simulink model "testrig_Bus_Makhulu_Parts"  (R2026a)
settings: Solver=VariableStepAuto  EnableMultiTasking=on
undefined symbols (not defined in the file): X, Y, Z
libraries: sm_lib x9, Bus_Makhulu_Parts x6, Passenger_Human x4, nesl_utility x1
Description:
  | Copyright 2020-2026 The MathWorks, Inc.
settings Model: Creator=smiller  LastModifiedBy=smiller
settings DataIOCC: SignalLoggingName=logsout_testrig_Bus_Makhulu_Parts
settings SimscapeCC: SimscapeNominalValues="[{\"value\":\"10\",\"unit\":\"V\"},{\"value\":\"1\",\"unit\":\"A\"},{\"value\":\"10\",\"unit\":\"N*m\"},{\"value\":\"10\",\"unit\":\"bar\"},{\"value\":\"100\",\"unit\":\"kJ/kg\"},{\"value\":\"1\",\"unit\":\"kW\"},{\"value\":\"300\",\"unit\":\"K\"},{\"value\":\"100\",\"unit\":\"cm^3/s\"},{\"value\":\"1\",\"unit\":\"kN\"},{\"value\":\"1\",\"unit\":\"g/cm^3\"},{\"value\":\"1\",\"unit\":\"l\"},{\"value\":\"1\",\"unit\":\"cm^2\"},{\"value\":\"60\",\"unit\":\"Hz\"}]"  SimscapeLogName=simlog_testrig_Bus_Makhulu_Parts
settings ConfigurationSet: Description=SimMechanics 2G
settings ExplorerConfigSet: InternalSimMechanicsExplorerSettings="<ExplorerConfiguration><canonicalview>default</canonicalview><AnimationSetting><BasePlaybackSpeed>1.0</BasePlaybackSpeed><PlaybackSpeedFactor>1.0</PlaybackSpeedFactor></AnimationSetting><TilePanel><TileInfo><Tiles Columns=\"4\" Count=\"6\" Rows=\"3\"><Column Weight=\"0.3469\"/><Column Weight=\"0.3469\"/><Column Weight=\"0.1531\"/><Column Weight=\"0.1531\"/><Row Weight=\"0.5025\"/><Row Weight=\"0.2487\"/><Row Weight=\"0.2487\"/><Tile Height=\"1\" Width=\"1\" X=\"0\" Y=\"0\"/><Tile Height=\"1\" Width=\"1\" X=\"1\" Y=\"0\"/><Tile Height=\"1\" Width=\"2\" X=\"0\" Y=\"1\"/><Tile Height=\"1\" Width=\"2\" X=\"0\" Y=\"2\"/><Tile Height=\"3\" Width=\"1\" X=\"2\" Y=\"0\"/><Tile Height=\"3\" Width=\"1\" X=\"3\" Y=\"0\"/></Tiles></TileInfo><SceneInfo><SceneViewer><BGColor><R>1</R><G>1</G><B>1</B></BGColor><Camera><DoPerspective>off</DoPerspective><Position><X>2.89597907673196531</X><Y>-0.00109799404478061469</Y><Z>1.33429143595940403</Z></Position><Center><X>-3.84443919785476673</X><Y>-0.00109799404478061469</Y><Z>1.33429143595940403</Z></Center><Up><X>-0</X><Y>0</Y><Z>1</Z></Up><ViewLimDist>1</ViewLimDist><YLim>1.37425733566284181</YLim><XLim>1.46067108293575876</XLim></Camera></SceneViewer><SceneViewer><BGColor><R>1</R><G>1</G><B>1</B></BGColor><Camera><DoPerspective>off</DoPerspective><Position><X>-10.8501736304465091</X><Y>-0.00109795652245203712</Y><Z>1.33429143595940225</Z></Position><Center><X>-3.84443855103689636</X><Y>-0.00109795652245203712</Y><Z>1.33429143595940225</Z></Center><Up><X>0</X><Y>0</Y><Z>1</Z></Up><ViewLimDist>1</ViewLimDist><YLim>1.37425733566284181</YLim><XLim>1.46067108293575876</XLim></Camera></SceneViewer><SceneViewer><BGColor><R>1</R><G>1</G><B>1</B></BGColor><Camera><DoPerspective>off</DoPerspective><Position><X>-3.84443881153779143</X><Y>-6.9199634574691915</Y><Z>1.33429143595940314</Z></Position><Center><X>-3.84443881153779143</X><Y>-0.00109763641691196234</Y><Z>1.33429143595940314</Z></Center><Up><X>0</X><Y>-0</Y><Z>1</Z></Up><ViewLimDist>1</ViewLimDist><YLim>1.37425733566284181</YLim><XLim>6.00243803221332239</XLim></Camera></SceneViewer><SceneViewer><BGColor><R>1</R><G>1</G><B>1</B></BGColor><Camera><DoPerspective>off</DoPerspective><Position><X>-3.84443881153779055</X><Y>6.9177671418572757</Y><Z>1.33429143595940136</Z></Position><Center><X>-3.84443881153779055</X><Y>-0.00109815741870300521</Y><Z>1.33429143595940136</Z></Center><Up><X>0</X><Y>0</Y><Z>1</Z></Up><ViewLimDist>1</ViewLimDist><YLim>1.37425733566284181</YLim><XLim>6.00243803221332239</XLim></Camera></SceneViewer><SceneViewer><BGColor><R>1</R><G>1</G><B>1</B></BGColor><Camera><DoPerspective>off</DoPerspective><Position><X>-3.84496310619994697</X><Y>0.00593013000974051963</Y><Z>8.58263582377032996</Z></Position><Center><X>-3.84496310619994697</X><Y>0.00593013000974051963</Y><Z>1.33429140250232159</Z></Center><Up><X>0.999999127014181366</X><Y>-0.00132135191201654401</Y><Z>0</Z></Up><ViewLimDist>1</ViewLimDist><YLim>5.96790659427642822</YLim><XLim>1.37351820109477596</XLim></Camera></SceneViewer><SceneViewer><BGColor><R>1</R><G>1</G><B>1</B></BGColor><Camera><DoPerspective>off</DoPerspective><Position><X>-3.84487511554848593</X><Y>-0.0069608981245425916</Y><Z>-5.25447968591559</Z></Position><Center><X>-3.84487511554848593</X><Y>-0.0069608981245425916</Y><Z>1.3342916573167356</Z></Center><Up><X>0.999999392465900749</X><Y>0.00110230115204205253</Y><Z>0</Z></Up><ViewLimDist>1</ViewLimDist><YLim>5.96775483131408713</YLim><XLim>1.37348327273459891</XLim></Camera></SceneViewer></SceneInfo></TilePanel><MechEditorPanel><Cameras/><GfxPanelCameraMap/><VideoCreator><PlaybackSpeedRatio>1.0</PlaybackSpeedRatio><FrameRate>30</FrameRate><VideoFormat>Motion JPEG AVI</VideoFormat><FrameSize>auto</FrameSize></VideoCreator></MechEditorPanel></ExplorerConfiguration>"

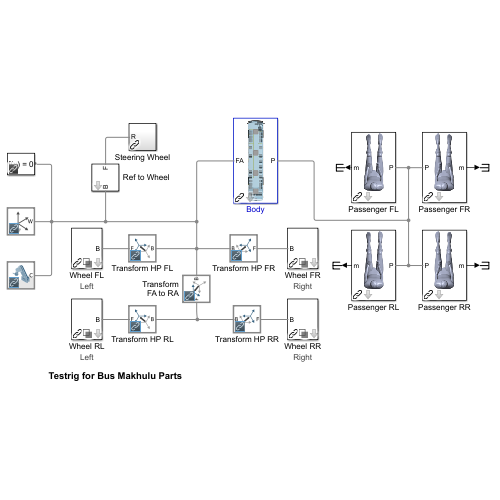
[thumbnail: Simulink's stored preview of the top-level diagram]
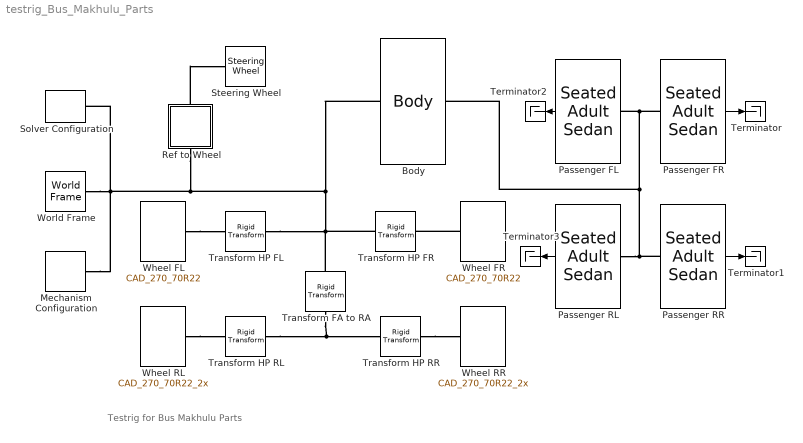
== system testrig_Bus_Makhulu_Parts ==
  note: Testrig for Bus Makhulu Parts
  Body : Bus_Makhulu_Parts/Body  body_offset=[0 0 0]  body_orient=[0 0 0]  body_clr=[0.55 0.85 1]  body_opc=1  glass_opc=BodyGeometry.GlassOpacity.Value
  Mechanism Configuration : sm_lib/Utilities/Mechanism Configuration  UniformGravity=Constant  GravityVector=[0 0 -9.80665]  GravityVectorUnits=m/s^2  LinearizationDelta=0.001  JointModeTransitionNonlinearIterations=2
  Passenger FL : Passenger_Human/Seated Adult Sedan  VariantControl=Variant1  hp_human=[-0.47 0.6 1.34]  rpy_human=[0 15 -90]  rho_human=Vehicle.Chassis.Body.Passenger.FL.rho.Value  human_clr=[0.792156862745098 0.819607843137255 0.933333333333333]  human_opc=1
  Passenger FR : Passenger_Human/Seated Adult Sedan  VariantControl=Variant1  hp_human=[-0.98 -0.6 1.34]  rpy_human=[0 15 90]  rho_human=Vehicle.Chassis.Body.Passenger.FL.rho.Value  human_clr=[0.792156862745098 0.819607843137255 0.933333333333333]  human_opc=1
  Passenger RL : Passenger_Human/Seated Adult Sedan  VariantControl=Variant1  hp_human=[-2.03 0.755 1.2]  rpy_human=[0 15 180]  rho_human=Vehicle.Chassis.Body.Passenger.FL.rho.Value  human_clr=[0.792156862745098 0.819607843137255 0.933333333333333]  human_opc=1
  Passenger RR : Passenger_Human/Seated Adult Sedan  VariantControl=Variant1  hp_human=[-3.05 -0.77 1.2]  rpy_human=[0 15 0]  rho_human=Vehicle.Chassis.Body.Passenger.FL.rho.Value  human_clr=[0.792156862745098 0.819607843137255 0.933333333333333]  human_opc=1
  Ref to Wheel : Subsystem  mask{hp_wheel=[1.2610308+0.01 0.55801 1.2685808], wheel_axis_incl=45.2*pi/180}
      mask prompts: hp_wheel "HP Steering Wheel [x y z] (m)"; wheel_axis_incl "Steering Inclination Angle (rad)"
  Solver Configuration : nesl_utility/Solver Configuration  PhysicalDomain=network_engine_domain  SubClassName=solver  LeftPortType=input  RightPortType=generic  Tones=[]  Harmonics=[]  SimulateNoise=off  Profile=off  UseLocalSampling=off  EnableSwitchedLinearOptims=on  FrequencyDomain=off  UseCCode=off  RelTol=0.001  AbsTol=1e-06  MinStep=1e-09  ToWorkspace=off  RevertToSquareIcSolve=off  NumHomotopyIterations=100  PhasorMode=off  PhasorModeNumHarmonics=1  ConsistencySolver=NEWTON_FTOL  CanonicalOrdering=UNORDERED  OptimizeIntermediates=UNOPTIMIZED  IndexReductionMethod=DerivativeReplacement  DoDC=off  ResidualTolerance=1e-09  ConsistencyTolSource=GLOBAL  ConsistencyAbsTol=0.001  ConsistencyRelTol=0.001  ConsistencyTolFactor=0.001  UseLocalSolver=off  LocalSolverChoice=NE_BACKWARD_EULER_ADVANCER  ResolveIndetEquations=on  FunctionEvalNumThread=1  LocalSolverSampleTime=0.001  DoFixedCost=off  MaxNonlinIter=3  MaxModeIter=2  ComputeImpulses=off  ImpulseIterations=2  LinearAlgebra=Sparse  LinearAlgebraNumThread=0  EquationFormulation=NE_TIME_EF  DelaysMemoryBudget=1024  AutomaticFiltering=on  FilteringTimeConstant=0.001  PartitionStorageMethod=AS_NEEDED  PartitionMemoryBudget=1024  PartitionMethod=FAST  MultibodyUseLocalSolver=off  MultibodyLocalSolverChoice=ODE1  MultibodyLocalSolverSampleTime=0.001
  Steering Wheel : Bus_Makhulu_Parts/Steering Wheel  SystemSampleTime=-1  VariantActivationTime=update diagram  EmptyChoice=off  PassThrough=off  PassThroughVariantControl=(default)  EmptyChoiceVariantControl=(default)  AllowFlexibleInterface=on  Latency=0  AutoFrameSizeCalculation=off
  Terminator{,1..3} (4 alike) : Terminator
  Transform FA to RA : sm_lib/Frames and Transforms/Rigid Transform  RotationMethod=None  FollAlignAxisA=+X  BaseAlignAxisA=+Y  FollAlignAxisB=+Y  BaseAlignAxisB=+Z  RotationStandardAxis=+Z  RotationAngle=0.0  RotationAngleUnits=deg  RotationArbitraryAxis=[0 0 1]  RotationSequenceAxes=FollowerAxes  RotationSequence=XYX  RotationSequenceAngles=[0 0 0]  RotationSequenceAnglesUnits=deg  RotationMatrix=[1 0 0; 0 1 0; 0 0 1]  Quaternion=[1 0 0 0]  TranslationMethod=StandardAxis  TranslationCartesianOffset=[0 0 0]  TranslationCartesianOffsetUnits=m  TranslationStandardAxis=+X  TranslationStandardOffset=-6.781616  TranslationStandardOffsetUnits=m  TranslationROffset=0  TranslationROffsetUnits=m  TranslationThetaOffset=0  TranslationThetaOffsetUnits=deg  TranslationZOffset=0  TranslationZOffsetUnits=m
  Transform HP FL : sm_lib/Frames and Transforms/Rigid Transform  RotationMethod=StandardAxis  FollAlignAxisA=+X  BaseAlignAxisA=+Y  FollAlignAxisB=+Y  BaseAlignAxisB=+Z  RotationStandardAxis=+X  RotationAngle=-90  RotationAngleUnits=deg  RotationArbitraryAxis=[0 0 1]  RotationSequenceAxes=FollowerAxes  RotationSequence=XYX  RotationSequenceAngles=[0 0 0]  RotationSequenceAnglesUnits=deg  RotationMatrix=[1 0 0; 0 1 0; 0 0 1]  Quaternion=[1 0 0 0]  TranslationMethod=Cartesian  TranslationCartesianOffset=[0 0.9829099 0.4613615]  TranslationCartesianOffsetUnits=m  TranslationStandardAxis=+Z  TranslationStandardOffset=0  TranslationStandardOffsetUnits=m  TranslationROffset=0  TranslationROffsetUnits=m  TranslationThetaOffset=0  TranslationThetaOffsetUnits=deg  TranslationZOffset=0  TranslationZOffsetUnits=m
  Transform HP FR : sm_lib/Frames and Transforms/Rigid Transform  RotationMethod=StandardAxis  FollAlignAxisA=+X  BaseAlignAxisA=+Y  FollAlignAxisB=+Y  BaseAlignAxisB=+Z  RotationStandardAxis=+X  RotationAngle=-90  RotationAngleUnits=deg  RotationArbitraryAxis=[0 0 1]  RotationSequenceAxes=FollowerAxes  RotationSequence=XYX  RotationSequenceAngles=[0 0 0]  RotationSequenceAnglesUnits=deg  RotationMatrix=[1 0 0; 0 1 0; 0 0 1]  Quaternion=[1 0 0 0]  TranslationMethod=Cartesian  TranslationCartesianOffset=[0 -0.9829099 0.4613615]  TranslationCartesianOffsetUnits=m  TranslationStandardAxis=+Z  TranslationStandardOffset=0  TranslationStandardOffsetUnits=m  TranslationROffset=0  TranslationROffsetUnits=m  TranslationThetaOffset=0  TranslationThetaOffsetUnits=deg  TranslationZOffset=0  TranslationZOffsetUnits=m
  Transform HP RL : sm_lib/Frames and Transforms/Rigid Transform  RotationMethod=StandardAxis  FollAlignAxisA=+X  BaseAlignAxisA=+Y  FollAlignAxisB=+Y  BaseAlignAxisB=+Z  RotationStandardAxis=+X  RotationAngle=-90  RotationAngleUnits=deg  RotationArbitraryAxis=[0 0 1]  RotationSequenceAxes=FollowerAxes  RotationSequence=XYX  RotationSequenceAngles=[0 0 0]  RotationSequenceAnglesUnits=deg  RotationMatrix=[1 0 0; 0 1 0; 0 0 1]  Quaternion=[1 0 0 0]  TranslationMethod=Cartesian  TranslationCartesianOffset="[0 0.838344+0.1359705  0.4613615]"  TranslationCartesianOffsetUnits=m  TranslationStandardAxis=+Z  TranslationStandardOffset=0  TranslationStandardOffsetUnits=m  TranslationROffset=0  TranslationROffsetUnits=m  TranslationThetaOffset=0  TranslationThetaOffsetUnits=deg  TranslationZOffset=0  TranslationZOffsetUnits=m
  Transform HP RR : sm_lib/Frames and Transforms/Rigid Transform  RotationMethod=StandardAxis  FollAlignAxisA=+X  BaseAlignAxisA=+Y  FollAlignAxisB=+Y  BaseAlignAxisB=+Z  RotationStandardAxis=+X  RotationAngle=-90  RotationAngleUnits=deg  RotationArbitraryAxis=[0 0 1]  RotationSequenceAxes=FollowerAxes  RotationSequence=XYX  RotationSequenceAngles=[0 0 0]  RotationSequenceAnglesUnits=deg  RotationMatrix=[1 0 0; 0 1 0; 0 0 1]  Quaternion=[1 0 0 0]  TranslationMethod=Cartesian  TranslationCartesianOffset=[0 -0.838344-0.1359705 0.4613615]  TranslationCartesianOffsetUnits=m  TranslationStandardAxis=+Z  TranslationStandardOffset=0  TranslationStandardOffsetUnits=m  TranslationROffset=0  TranslationROffsetUnits=m  TranslationThetaOffset=0  TranslationThetaOffsetUnits=deg  TranslationZOffset=0  TranslationZOffsetUnits=m
  Wheel FL : Bus_Makhulu_Parts/CAD_270_70R22  LabelModeActiveChoice=Left  popup_leftRight=Left  mass_tire=10  mass_rim=0  tire_inertia=[1 2]  rim_inertia=[0 0]  offset_cg=[0 0 0]
      settings: AttributesFormatString=%<LabelModeActiveChoice>
  Wheel FR : Bus_Makhulu_Parts/CAD_270_70R22  LabelModeActiveChoice=Right  popup_leftRight=Right  mass_tire=10  mass_rim=0  tire_inertia=[1 2]  rim_inertia=[0 0]  offset_cg=[0 0 0]
      settings: AttributesFormatString=%<LabelModeActiveChoice>
  Wheel RL : Bus_Makhulu_Parts/CAD_270_70R22_2x  LabelModeActiveChoice=Left  popup_leftRight=Left  mass_tire=10  mass_rim=0  tire_inertia=[1 2]  rim_inertia=[0 0]  offset_cg=[0 0 0]
      settings: AttributesFormatString=%<LabelModeActiveChoice>
  Wheel RR : Bus_Makhulu_Parts/CAD_270_70R22_2x  LabelModeActiveChoice=Right  popup_leftRight=Right  mass_tire=10  mass_rim=0  tire_inertia=[1 2]  rim_inertia=[0 0]  offset_cg=[0 0 0]
      settings: AttributesFormatString=%<LabelModeActiveChoice>
  World Frame : sm_lib/Frames and Transforms/World Frame
  wires:
  Passenger FR/1 -> Terminator/1
  Passenger RR/1 -> Terminator1/1
  Passenger FL/1 -> Terminator2/1
  Passenger RL/1 -> Terminator3/1
  connections:
  Ref to Wheel/RConn1 -- Steering Wheel/LConn1
  Wheel RL/LConn1 -- Transform HP RL/RConn1
  Transform HP RL/LConn1 -- Transform HP RR/LConn1 -- Transform FA to RA/RConn1
  Transform HP RR/RConn1 -- Wheel RR/LConn1
  Wheel FL/LConn1 -- Transform HP FL/RConn1
  Wheel FR/LConn1 -- Transform HP FR/RConn1
  Mechanism Configuration/RConn1 -- Solver Configuration/RConn1 -- Ref to Wheel/LConn1 -- Body/RConn1 -- Transform FA to RA/LConn1 -- Transform HP FR/LConn1 -- Transform HP FL/LConn1 -- World Frame/RConn1
  Passenger RL/LConn1 -- Body/LConn1 -- Passenger FL/LConn1 -- Passenger FR/LConn1 -- Passenger RR/LConn1

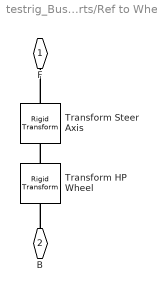
== system testrig_Bus_Makhulu_Parts/Ref to Wheel ==
  Transform HP Wheel : sm_lib/Frames and Transforms/Rigid Transform  RotationMethod=None  FollAlignAxisA=+X  BaseAlignAxisA=+Y  FollAlignAxisB=+Y  BaseAlignAxisB=+Z  RotationStandardAxis=+Z  RotationAngle=0.0  RotationAngleUnits=deg  RotationArbitraryAxis=[0 0 1]  RotationSequenceAxes=FollowerAxes  RotationSequence=XYX  RotationSequenceAngles=[0 0 0]  RotationSequenceAnglesUnits=deg  RotationMatrix=[1 0 0; 0 1 0; 0 0 1]  Quaternion=[1 0 0 0]  TranslationMethod=Cartesian  TranslationCartesianOffset=hp_wheel  TranslationCartesianOffsetUnits=m  TranslationStandardAxis=+Z  TranslationStandardOffset=0  TranslationStandardOffsetUnits=m  TranslationROffset=0  TranslationROffsetUnits=m  TranslationThetaOffset=0  TranslationThetaOffsetUnits=deg  TranslationZOffset=0  TranslationZOffsetUnits=m
  Transform Steer Axis : sm_lib/Frames and Transforms/Rigid Transform  RotationMethod=StandardAxis  FollAlignAxisA=+X  BaseAlignAxisA=+Y  FollAlignAxisB=+Y  BaseAlignAxisB=+Z  RotationStandardAxis=+Y  RotationAngle=-pi/2+wheel_axis_incl  RotationAngleUnits=rad  RotationArbitraryAxis=[0 0 1]  RotationSequenceAxes=FollowerAxes  RotationSequence=XYX  RotationSequenceAngles=[0 0 0]  RotationSequenceAnglesUnits=deg  RotationMatrix=[1 0 0; 0 1 0; 0 0 1]  Quaternion=[1 0 0 0]  TranslationMethod=None  TranslationCartesianOffset=[0 0 0]  TranslationCartesianOffsetUnits=m  TranslationStandardAxis=+Z  TranslationStandardOffset=0  TranslationStandardOffsetUnits=m  TranslationROffset=0  TranslationROffsetUnits=m  TranslationThetaOffset=0  TranslationThetaOffsetUnits=deg  TranslationZOffset=0  TranslationZOffsetUnits=m
  F : PMIOPort  Side=Right
  B : PMIOPort  Port=2  Side=Left
  connections:
  Transform Steer Axis/RConn1 -- F/RConn1
  B/RConn1 -- Transform HP Wheel/LConn1
  Transform HP Wheel/RConn1 -- Transform Steer Axis/LConn1
